simulink model "PosCtrl_tune"  (R2020b)
settings: Solver=FixedStepAuto  StartTime=0.0  StopTime=inf  FixedStep=0.01  RelTol=1e-3
InitFcn:
  | Init_control;
values from neighbouring files (symbols this model uses):
  DEG2RAD = 0.0174533    [Init_control.m]
  Kd_PITCH_AngleRate = 0.001    [Init_control.m]
  Kd_ROLL_AngleRate = 0.001    [Init_control.m]
  Kd_YAW_AngleRate = 0.00    (= 0)    [Init_control.m]
  Ki_PITCH_AngleRate = 0.02    [Init_control.m]
  Ki_ROLL_AngleRate = 0.02    [Init_control.m]
  Ki_YAW_AngleRate = 0.01    [Init_control.m]
  Kp_PITCH_ANGLE = 6.5    [Init_control.m]
  Kp_PITCH_AngleRate = 0.1    [Init_control.m]
  Kp_ROLL_ANGLE = 6.5    [Init_control.m]
  Kp_ROLL_AngleRate = 0.1    [Init_control.m]
  Kp_YAW_ANGLE = 3    [Init_control.m]
  Kp_YAW_AngleRate = 0.5    [Init_control.m]
  Kpxp = 1.0    (= 1)    [Init_control.m]
  Kpyp = 1.0    (= 1)    [Init_control.m]
  Kpzp = 4.0    (= 4)    [Init_control.m]
  Kvxd = 0.01    [Init_control.m]
  Kvxi = 0.4    [Init_control.m]
  Kvxp = 2.5    [Init_control.m]
  Kvyd = 0.01    [Init_control.m]
  Kvyi = 0.4    [Init_control.m]
  Kvyp = 2.5    [Init_control.m]
  Kvzd = 0.005    [Init_control.m]
  Kvzi = 0.01    [Init_control.m]
  Kvzp = 0.45    [Init_control.m]
  MAX_CONTROL_ANGLE_PITCH = 35    [Init_control.m]
  MAX_CONTROL_ANGLE_RATE_PITCH = 220    [Init_control.m]
  MAX_CONTROL_ANGLE_RATE_ROLL = 220    [Init_control.m]
  MAX_CONTROL_ANGLE_RATE_Y = 200    [Init_control.m]
  MAX_CONTROL_ANGLE_ROLL = 35    [Init_control.m]
  MAX_CONTROL_VELOCITY_XY = 17.6    [Init_control.m]
  MAX_CONTROL_VELOCITY_Z = 5    [Init_control.m]
  MAX_MAN_THR = 0.9    [Init_control.m]
  ModelInit_AngEuler = [0, 0, 0]    [Init_control.m]
  ModelInit_PosE0 = [0, 0, 0]    [Init_control.m]
  ModelInit_Rads = sqrt((ModelParam_uavMass*ModelParam_envGravityAcc)/(4*ModelParam_rotorCt))    [Init_control.m]
  ModelInit_RateB = [0, 0, 0]    [Init_control.m]
  ModelInit_VelB = [0, 0, 0]    [Init_control.m]
  Saturation_I_ah = 3.43    [Init_control.m]
  Saturation_I_az = 5    [Init_control.m]
  Saturation_I_RP_Max = 0.3    [Init_control.m]
  Saturation_I_RP_Min = -0.3    [Init_control.m]
  Saturation_I_Y_Max = 0.2    [Init_control.m]
  Saturation_I_Y_Min = -0.2    [Init_control.m]
  THR_HOVER = (ModelInit_Rads-ModelParam_motorWb)/ModelParam_motorCr    [Init_control.m]
undefined symbols (not defined in the file or in its folder): DiscIntNeverNeededParam, ModelParam_envGravityAcc, ModelParam_motorCr, ModelParam_motorJm, ModelParam_motorT, ModelParam_motorWb, ModelParam_rotorCm, ModelParam_rotorCt, ModelParam_uavCCm, ModelParam_uavCd, ModelParam_uavJ, ModelParam_uavMass, ModelParam_uavR
libraries: simulink x24, slrealtimeutilitieslib x8, sharedutil x8, dspnetwork x8, aerolibanimutils x1
(part 1 of 3)
settings Model: Creator=wsh  LastModifiedBy=chenjiaqing
settings DataIOCC: ReturnWorkspaceOutputs=off
settings DebuggingCC: BusObjectLabelMismatch=error  ArithmeticOperatorsInVariantConditions=warning
settings SFSimCC: SimUseLocalCustomCode=off  CustomCodeUndefinedFunction=UseInterfaceOnly
settings RTWCC: RTWUseLocalCustomCode=off
settings CodeAppCC: StateflowObjectComments=on

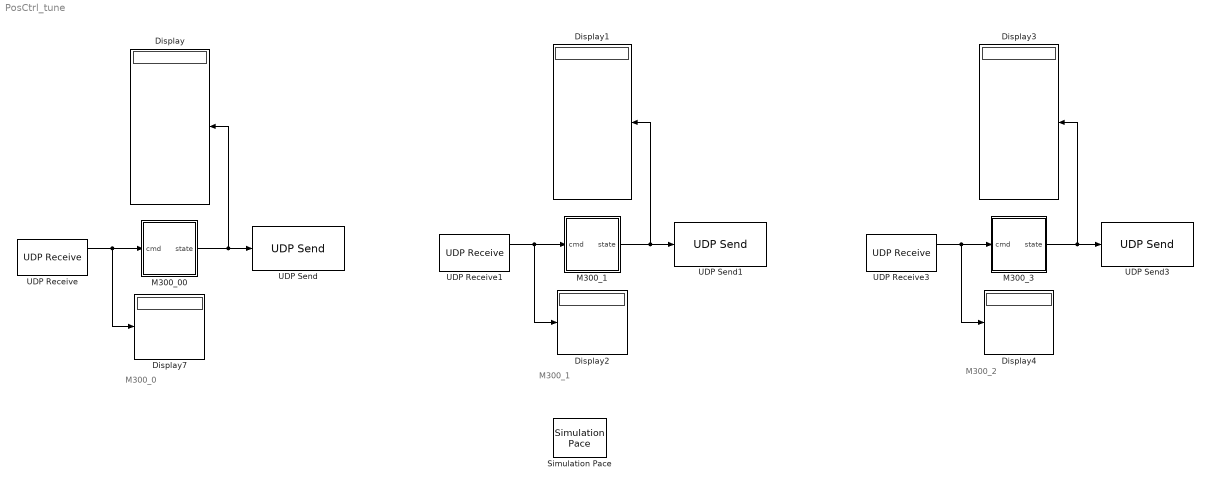
== system PosCtrl_tune ==
  note: M300_0
  note: M300_1
  note: M300_2
  Display{,1..4,7} (6 alike) : Display
      Display2 settings: Decimation=4
      Display4 settings: Decimation=4
      Display7 settings: Decimation=4
  M300_00 : Subsystem
  M300_1 : Subsystem
  M300_3 : Subsystem
  Simulation Pace : aerolibanimutils/Simulation Pace  SimulationPace=1  SleepMode=MATLAB Thread  OutputPaceError=off  SampleTime=-1
      settings: AttributesFormatString=%<SimulationPace> sec/sec
  UDP Receive : dspnetwork/UDP Receive  localURL='0.0.0.0'  localPort=udp_cmd0  remoteURL='127.0.0.1'  remotePort=-1  recvBufferSize=4  dims=4  signalDatatype=double  isComplex=off  isVarSize=off  showBlockingTime=off  blockingTime=0  sampletime=-1  blockPlatform=[]
  UDP Receive1 : dspnetwork/UDP Receive  localURL='0.0.0.0'  localPort=udp_cmd1  remoteURL='127.0.0.1'  remotePort=-1  recvBufferSize=4  dims=4  signalDatatype=double  isComplex=off  isVarSize=off  showBlockingTime=off  blockingTime=0  sampletime=-1  blockPlatform=[]
  UDP Receive3 : dspnetwork/UDP Receive  localURL='0.0.0.0'  localPort=udp_cmd2  remoteURL='127.0.0.1'  remotePort=-1  recvBufferSize=4  dims=4  signalDatatype=double  isComplex=off  isVarSize=off  showBlockingTime=off  blockingTime=0  sampletime=-1  blockPlatform=[]
  UDP Send : dspnetwork/UDP Send  remoteURL='127.0.0.1'  remotePort=udp_state0  localURL='0.0.0.0'  localPortSource=Automatically determine  localPort=25000  sendBufferSize=1  sampletime=-1  blockPlatform=[]  separateLengthPort=0
  UDP Send1 : dspnetwork/UDP Send  remoteURL='127.0.0.1'  remotePort=udp_state1  localURL='0.0.0.0'  localPortSource=Automatically determine  localPort=25000  sendBufferSize=1  sampletime=-1  blockPlatform=[]  separateLengthPort=0
  UDP Send3 : dspnetwork/UDP Send  remoteURL='127.0.0.1'  remotePort=udp_state2  localURL='0.0.0.0'  localPortSource=Automatically determine  localPort=25000  sendBufferSize=1  sampletime=-1  blockPlatform=[]  separateLengthPort=0
  wires:
  UDP Receive/1 -> Display7/1, M300_00/1(cmd)
  M300_00/1(state) -> UDP Send/1, Display/1
  UDP Receive1/1 -> Display2/1, M300_1/1(cmd)
  M300_1/1(state) -> UDP Send1/1, Display1/1
  UDP Receive3/1 -> Display4/1, M300_3/1(cmd)
  M300_3/1(state) -> UDP Send3/1, Display3/1

== system PosCtrl_tune/M300_00 ==
  cmd : Inport
  Byte Packing : slrealtimeutilitieslib/Byte Packing  MaskPackedDataType=double  MaskUnpackedDataTypes={'double','double','double','double','double','double','double','double','double','double'}  MaskAlignment=1
  Byte Unpacking : slrealtimeutilitieslib/Byte Unpacking  MaskUnpackedDataTypes={'double','double','double','double'}  MaskUnpackedDataSizes={[1],[1],[1],[1]}  MaskAlignment=1
      settings: SourceProductBaseCode=XP
  Constant : Constant  Value=0
  Control System : Subsystem
  Demux{,1..3,5..6} (6 alike) : Demux  Outputs=3
  Demux4 : Demux
  Quadcopter Dynamics : Subsystem
  Terminator{,1..5} (6 alike) : Terminator
  state : Outport
  wires:
  Quadcopter Dynamics/2(VelE) -> Demux5/1, Demux3/1  "VelE"
  Quadcopter Dynamics/4(AngRateB) -> Demux6/1, Demux/1  "AngRateB"
  Demux1/1 -> Byte Packing/4, Control System/11(roll)
  Demux2/1 -> Byte Packing/1, Control System/14(x)
  Demux1/2 -> Byte Packing/5, Control System/12(pitch)
  Demux1/3 -> Byte Packing/6, Control System/13(yaw)
  Demux4/2 -> Byte Packing/8
  Demux2/2 -> Control System/15(y), Byte Packing/2
  Constant/1 -> Control System/5(vxd), Control System/6(vyd), Control System/7(vzd)
  Quadcopter Dynamics/5(MotorRPMS) -> Demux4/1
  Demux2/3 -> Control System/16(z), Byte Packing/3
  Demux4/3 -> Byte Packing/7
  Quadcopter Dynamics/1(PosE) -> Demux2/1  "PosE"
  Demux4/4 -> Byte Packing/9
  Demux/3 -> Control System/10(r)
  Demux4/1 -> Byte Packing/10
  Quadcopter Dynamics/3(AngEuler) -> Demux1/1  "AngEular"
  Demux/1 -> Control System/8(p)
  Demux/2 -> Control System/9(q)
  Control System/1(PWM) -> Quadcopter Dynamics/1(inPWMs)
  Demux3/3 -> Control System/19(vz)
  Demux3/1 -> Control System/17(vx)
  Demux3/2 -> Control System/18(vy)
  cmd/1 -> Byte Unpacking/1
  Byte Packing/1 -> state/1
  Byte Unpacking/1 -> Control System/1(xd)
  Byte Unpacking/2 -> Control System/2(yd)
  Byte Unpacking/3 -> Control System/3(zd)
  Byte Unpacking/4 -> Control System/4(yaw_d)
  Demux5/1 -> Terminator/1
  Demux5/2 -> Terminator1/1
  Demux5/3 -> Terminator2/1
  Demux6/3 -> Terminator5/1
  Demux6/1 -> Terminator3/1
  Demux6/2 -> Terminator4/1

== system PosCtrl_tune/M300_1 ==
  cmd : Inport
  Byte Packing : slrealtimeutilitieslib/Byte Packing  MaskPackedDataType=double  MaskUnpackedDataTypes={'double','double','double','double','double','double','double','double','double','double'}  MaskAlignment=1
  Byte Unpacking : slrealtimeutilitieslib/Byte Unpacking  MaskUnpackedDataTypes={'double','double','double','double'}  MaskUnpackedDataSizes={[1],[1],[1],[1]}  MaskAlignment=1
      settings: SourceProductBaseCode=XP
  Constant : Constant  Value=0
  Control System : Subsystem
  Demux{,1..3,5..6} (6 alike) : Demux  Outputs=3
  Demux4 : Demux
  Quadcopter Dynamics : Subsystem
  Terminator{,1..5} (6 alike) : Terminator
  state : Outport
  wires:
  Quadcopter Dynamics/2(VelE) -> Demux5/1, Demux3/1  "VelE"
  Quadcopter Dynamics/4(AngRateB) -> Demux6/1, Demux/1  "AngRateB"
  Demux1/1 -> Byte Packing/4, Control System/11(roll)
  Demux2/1 -> Byte Packing/1, Control System/14(x)
  Demux1/2 -> Byte Packing/5, Control System/12(pitch)
  Demux1/3 -> Byte Packing/6, Control System/13(yaw)
  Demux4/2 -> Byte Packing/8
  Demux2/2 -> Control System/15(y), Byte Packing/2
  Constant/1 -> Control System/5(vxd), Control System/6(vyd), Control System/7(vzd)
  Quadcopter Dynamics/5(MotorRPMS) -> Demux4/1
  Demux2/3 -> Control System/16(z), Byte Packing/3
  Demux4/3 -> Byte Packing/7
  Quadcopter Dynamics/1(PosE) -> Demux2/1  "PosE"
  Demux4/4 -> Byte Packing/9
  Demux/3 -> Control System/10(r)
  Demux4/1 -> Byte Packing/10
  Quadcopter Dynamics/3(AngEuler) -> Demux1/1  "AngEular"
  Demux/1 -> Control System/8(p)
  Demux/2 -> Control System/9(q)
  Control System/1(PWM) -> Quadcopter Dynamics/1(inPWMs)
  Demux3/3 -> Control System/19(vz)
  Demux3/1 -> Control System/17(vx)
  Demux3/2 -> Control System/18(vy)
  cmd/1 -> Byte Unpacking/1
  Byte Packing/1 -> state/1
  Byte Unpacking/1 -> Control System/1(xd)
  Byte Unpacking/2 -> Control System/2(yd)
  Byte Unpacking/3 -> Control System/3(zd)
  Byte Unpacking/4 -> Control System/4(yaw_d)
  Demux5/1 -> Terminator/1
  Demux5/2 -> Terminator1/1
  Demux5/3 -> Terminator2/1
  Demux6/3 -> Terminator5/1
  Demux6/1 -> Terminator3/1
  Demux6/2 -> Terminator4/1

== system PosCtrl_tune/M300_3 ==
  cmd : Inport
  Byte Packing : slrealtimeutilitieslib/Byte Packing  MaskPackedDataType=double  MaskUnpackedDataTypes={'double','double','double','double','double','double','double','double','double','double'}  MaskAlignment=1
  Byte Unpacking : slrealtimeutilitieslib/Byte Unpacking  MaskUnpackedDataTypes={'double','double','double','double'}  MaskUnpackedDataSizes={[1],[1],[1],[1]}  MaskAlignment=1
      settings: SourceProductBaseCode=XP
  Constant : Constant  Value=0
  Control System : Subsystem
  Demux{,1..3,5..6} (6 alike) : Demux  Outputs=3
  Demux4 : Demux
  M300_2 : Subsystem  Commented=on
  Quadcopter Dynamics : Subsystem
  Terminator{,1..5} (6 alike) : Terminator
  UDP Receive2 : dspnetwork/UDP Receive  Commented=on  localURL='0.0.0.0'  localPort=udp_cmd2  remoteURL='127.0.0.1'  remotePort=-1  recvBufferSize=4  dims=4  signalDatatype=double  isComplex=off  isVarSize=off  showBlockingTime=off  blockingTime=0  sampletime=-1  blockPlatform=[]
  UDP Send2 : dspnetwork/UDP Send  Commented=on  remoteURL='127.0.0.1'  remotePort=udp_state2  localURL='0.0.0.0'  localPortSource=Automatically determine  localPort=25000  sendBufferSize=1  sampletime=-1  blockPlatform=[]  separateLengthPort=0
  state : Outport
  wires:
  Quadcopter Dynamics/2(VelE) -> Demux5/1, Demux3/1  "VelE"
  Quadcopter Dynamics/4(AngRateB) -> Demux6/1, Demux/1  "AngRateB"
  Demux1/1 -> Byte Packing/4, Control System/11(roll)
  Demux2/1 -> Byte Packing/1, Control System/14(x)
  Demux1/2 -> Byte Packing/5, Control System/12(pitch)
  Demux1/3 -> Byte Packing/6, Control System/13(yaw)
  Demux4/2 -> Byte Packing/8
  Demux2/2 -> Control System/15(y), Byte Packing/2
  Constant/1 -> Control System/5(vxd), Control System/6(vyd), Control System/7(vzd)
  Quadcopter Dynamics/5(MotorRPMS) -> Demux4/1
  Demux2/3 -> Control System/16(z), Byte Packing/3
  Demux4/3 -> Byte Packing/7
  Quadcopter Dynamics/1(PosE) -> Demux2/1  "PosE"
  Demux4/4 -> Byte Packing/9
  Demux/3 -> Control System/10(r)
  Demux4/1 -> Byte Packing/10
  Quadcopter Dynamics/3(AngEuler) -> Demux1/1  "AngEular"
  Demux/1 -> Control System/8(p)
  Demux/2 -> Control System/9(q)
  Control System/1(PWM) -> Quadcopter Dynamics/1(inPWMs)
  Demux3/3 -> Control System/19(vz)
  Demux3/1 -> Control System/17(vx)
  Demux3/2 -> Control System/18(vy)
  cmd/1 -> Byte Unpacking/1
  Byte Packing/1 -> state/1
  Byte Unpacking/1 -> Control System/1(xd)
  Byte Unpacking/2 -> Control System/2(yd)
  Byte Unpacking/3 -> Control System/3(zd)
  Byte Unpacking/4 -> Control System/4(yaw_d)
  Demux5/1 -> Terminator/1
  Demux5/2 -> Terminator1/1
  Demux5/3 -> Terminator2/1
  Demux6/3 -> Terminator5/1
  Demux6/1 -> Terminator3/1
  Demux6/2 -> Terminator4/1
  M300_2/1(state) -> UDP Send2/1
  UDP Receive2/1 -> M300_2/1(cmd)

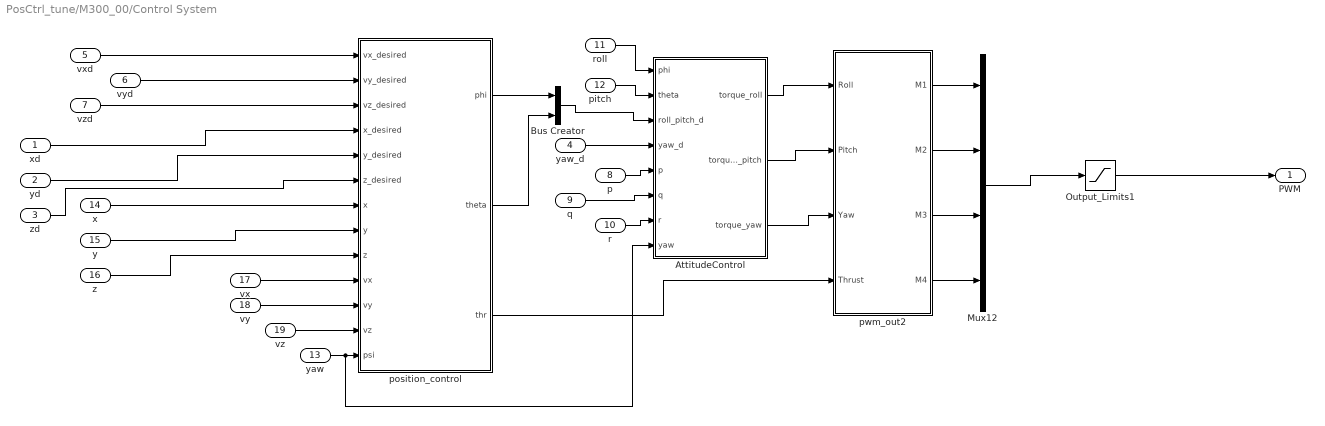
== system PosCtrl_tune/M300_00/Control System ==
  xd : Inport
  yd : Inport  Port=2
  zd : Inport  Port=3
  yaw_d : Inport  Port=4
  vxd : Inport  Port=5
  vyd : Inport  Port=6
  vzd : Inport  Port=7
  p : Inport  Port=8  PortDimensions=1
  q : Inport  Port=9  PortDimensions=1
  r : Inport  Port=10  PortDimensions=1
  roll : Inport  Port=11  PortDimensions=1
  pitch : Inport  Port=12  PortDimensions=1
  yaw : Inport  Port=13  PortDimensions=1
  x : Inport  Port=14
  y : Inport  Port=15
  z : Inport  Port=16
  vx : Inport  Port=17
  vy : Inport  Port=18
  vz : Inport  Port=19
  AttitudeControl : Subsystem
  Bus Creator : BusCreator  Inputs=2
  Mux12 : Mux
  Output_Limits1 : Saturate  UpperLimit=2000  LowerLimit=1000
  position_control : Subsystem
  pwm_out2 : MATLAB Function  SystemSampleTime=0.004
  PWM : Outport  VectorParamsAs1DForOutWhenUnconnected=off
  wires:
  Mux12/1 -> Output_Limits1/1
  AttitudeControl/2(torque_pitch) -> pwm_out2/2(Pitch)
  AttitudeControl/1(torque_roll) -> pwm_out2/1(Roll)
  pwm_out2/1(M1) -> Mux12/1
  pwm_out2/3(M3) -> Mux12/3
  pwm_out2/2(M2) -> Mux12/2
  AttitudeControl/3(torque_yaw) -> pwm_out2/3(Yaw)
  yaw_d/1 -> AttitudeControl/4(yaw_d)
  p/1 -> AttitudeControl/5(p)
  pwm_out2/4(M4) -> Mux12/4
  roll/1 -> AttitudeControl/1(phi)
  pitch/1 -> AttitudeControl/2(theta)
  position_control/1(phi) -> Bus Creator/1
  position_control/2(theta) -> Bus Creator/2
  Bus Creator/1 -> AttitudeControl/3(roll_pitch_d)
  position_control/3(thr) -> pwm_out2/4(Thrust)
  vxd/1 -> position_control/1(vx_desired)
  vyd/1 -> position_control/2(vy_desired)
  vzd/1 -> position_control/3(vz_desired)
  x/1 -> position_control/7(x)
  y/1 -> position_control/8(y)
  z/1 -> position_control/9(z)
  vx/1 -> position_control/10(vx)
  vy/1 -> position_control/11(vy)
  vz/1 -> position_control/12(vz)
  yaw/1 -> AttitudeControl/8(yaw), position_control/13(psi)
  Output_Limits1/1 -> PWM/1
  r/1 -> AttitudeControl/7(r)
  q/1 -> AttitudeControl/6(q)
  xd/1 -> position_control/4(x_desired)
  yd/1 -> position_control/5(y_desired)
  zd/1 -> position_control/6(z_desired)

== system PosCtrl_tune/M300_00/Quadcopter Dynamics ==
  note: 输入为1000至2000的PWM信号，
      | 需要归一化为0~1。
  inPWMs : Inport
  Constant2 : Constant  Value=[1000,1000,1000,1000]
  Demux2 : Demux
  Gain : Gain  Gain=30/pi
  Gain1 : Gain  Gain=1/1000
  Gain2 : Gain  Gain=-1
  Gain3 : Gain  Gain=10
  Gain4 : Gain  Gain=-1
  Gain5 : Gain
  Gain6 : Gain
  Mux : Mux
  Product1 : Product
  Saturation : Saturate  UpperLimit=1  LowerLimit=0
  Sum : Sum  Inputs=|+-
  g : Constant  Value=[0,0,ModelParam_envGravityAcc]
  mass : Constant  Value=ModelParam_uavMass
  六自由度模型 : Subsystem
  控制效果模型 : Subsystem
  电机动态模型 : Subsystem
  PosE : Outport  VectorParamsAs1DForOutWhenUnconnected=off
  VelE : Outport  Port=2  VectorParamsAs1DForOutWhenUnconnected=off
  AngEuler : Outport  Port=3  VectorParamsAs1DForOutWhenUnconnected=off
  AngRateB : Outport  Port=4  VectorParamsAs1DForOutWhenUnconnected=off
  MotorRPMS : Outport  Port=5  VectorParamsAs1DForOutWhenUnconnected=off
  wires:
  Saturation/1 -> 电机动态模型/1(inPWMs)
  六自由度模型/6("p,q,r ") -> 控制效果模型/5(p.q,r), AngRateB/1
  mass/1 -> Product1/1
  六自由度模型/4(DCM) -> 控制效果模型/3(DCM)
  电机动态模型/1(MotorRads) -> Gain/1, 控制效果模型/1(MotorRads)
  Gain1/1 -> Saturation/1
  六自由度模型/2(ve) -> VelE/1
  Sum/1 -> Gain1/1
  Product1/1 -> 控制效果模型/2(mg)
  六自由度模型/5("vb ") -> 控制效果模型/4(Vb)
  六自由度模型/1("xe ") -> PosE/1
  六自由度模型/3(Euler) -> AngEuler/1
  控制效果模型/1(Mb) -> 六自由度模型/1(Mb)
  inPWMs/1 -> Sum/1
  控制效果模型/2(Fb) -> 六自由度模型/2(f)
  Constant2/1 -> Sum/2
  g/1 -> Product1/2
  Demux2/3 -> Gain4/1
  Demux2/4 -> Gain6/1
  Gain2/1 -> Mux/1
  Gain4/1 -> Mux/3
  Gain6/1 -> Mux/4
  Mux/1 -> Gain3/1
  Demux2/1 -> Gain2/1
  Gain5/1 -> Mux/2
  Demux2/2 -> Gain5/1
  Gain/1 -> Demux2/1
  Gain3/1 -> MotorRPMS/1

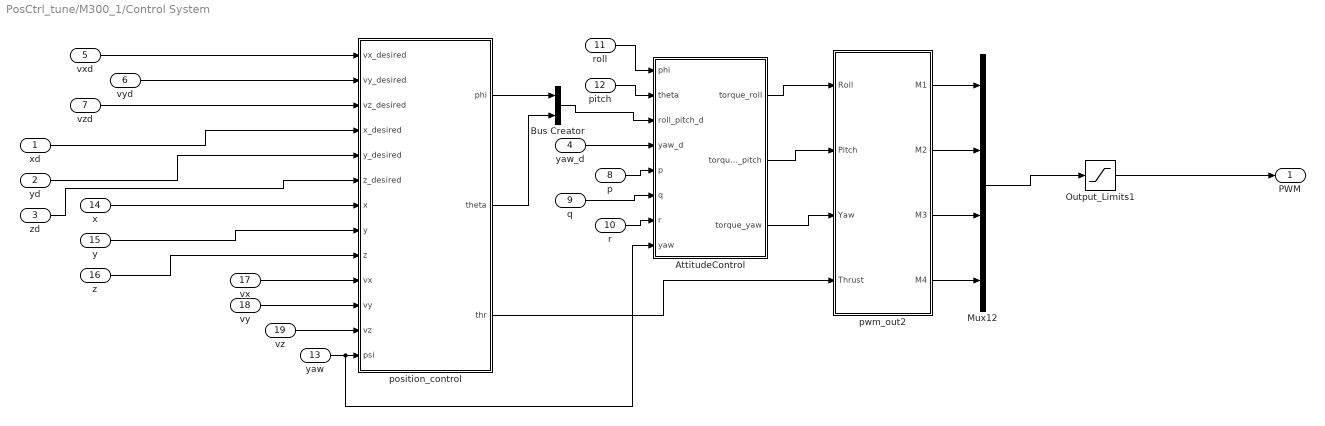
== system PosCtrl_tune/M300_1/Control System ==
  xd : Inport
  yd : Inport  Port=2
  zd : Inport  Port=3
  yaw_d : Inport  Port=4
  vxd : Inport  Port=5
  vyd : Inport  Port=6
  vzd : Inport  Port=7
  p : Inport  Port=8  PortDimensions=1
  q : Inport  Port=9  PortDimensions=1
  r : Inport  Port=10  PortDimensions=1
  roll : Inport  Port=11  PortDimensions=1
  pitch : Inport  Port=12  PortDimensions=1
  yaw : Inport  Port=13  PortDimensions=1
  x : Inport  Port=14
  y : Inport  Port=15
  z : Inport  Port=16
  vx : Inport  Port=17
  vy : Inport  Port=18
  vz : Inport  Port=19
  AttitudeControl : Subsystem
  Bus Creator : BusCreator  Inputs=2
  Mux12 : Mux
  Output_Limits1 : Saturate  UpperLimit=2000  LowerLimit=1000
  position_control : Subsystem
  pwm_out2 : MATLAB Function  SystemSampleTime=0.004
  PWM : Outport  VectorParamsAs1DForOutWhenUnconnected=off
  wires:
  Mux12/1 -> Output_Limits1/1
  AttitudeControl/2(torque_pitch) -> pwm_out2/2(Pitch)
  AttitudeControl/1(torque_roll) -> pwm_out2/1(Roll)
  pwm_out2/1(M1) -> Mux12/1
  pwm_out2/3(M3) -> Mux12/3
  pwm_out2/2(M2) -> Mux12/2
  AttitudeControl/3(torque_yaw) -> pwm_out2/3(Yaw)
  yaw_d/1 -> AttitudeControl/4(yaw_d)
  p/1 -> AttitudeControl/5(p)
  pwm_out2/4(M4) -> Mux12/4
  roll/1 -> AttitudeControl/1(phi)
  pitch/1 -> AttitudeControl/2(theta)
  position_control/1(phi) -> Bus Creator/1
  position_control/2(theta) -> Bus Creator/2
  Bus Creator/1 -> AttitudeControl/3(roll_pitch_d)
  position_control/3(thr) -> pwm_out2/4(Thrust)
  vxd/1 -> position_control/1(vx_desired)
  vyd/1 -> position_control/2(vy_desired)
  vzd/1 -> position_control/3(vz_desired)
  x/1 -> position_control/7(x)
  y/1 -> position_control/8(y)
  z/1 -> position_control/9(z)
  vx/1 -> position_control/10(vx)
  vy/1 -> position_control/11(vy)
  vz/1 -> position_control/12(vz)
  yaw/1 -> AttitudeControl/8(yaw), position_control/13(psi)
  Output_Limits1/1 -> PWM/1
  r/1 -> AttitudeControl/7(r)
  q/1 -> AttitudeControl/6(q)
  xd/1 -> position_control/4(x_desired)
  yd/1 -> position_control/5(y_desired)
  zd/1 -> position_control/6(z_desired)

== system PosCtrl_tune/M300_1/Quadcopter Dynamics ==
  note: 输入为1000至2000的PWM信号，
      | 需要归一化为0~1。
  inPWMs : Inport
  Constant2 : Constant  Value=[1000,1000,1000,1000]
  Demux2 : Demux
  Gain : Gain  Gain=30/pi
  Gain1 : Gain  Gain=1/1000
  Gain2 : Gain  Gain=-1
  Gain3 : Gain  Gain=10
  Gain4 : Gain  Gain=-1
  Gain5 : Gain
  Gain6 : Gain
  Mux : Mux
  Product1 : Product
  Saturation : Saturate  UpperLimit=1  LowerLimit=0
  Sum : Sum  Inputs=|+-
  g : Constant  Value=[0,0,ModelParam_envGravityAcc]
  mass : Constant  Value=ModelParam_uavMass
  六自由度模型 : Subsystem
  控制效果模型 : Subsystem
  电机动态模型 : Subsystem
  PosE : Outport  VectorParamsAs1DForOutWhenUnconnected=off
  VelE : Outport  Port=2  VectorParamsAs1DForOutWhenUnconnected=off
  AngEuler : Outport  Port=3  VectorParamsAs1DForOutWhenUnconnected=off
  AngRateB : Outport  Port=4  VectorParamsAs1DForOutWhenUnconnected=off
  MotorRPMS : Outport  Port=5  VectorParamsAs1DForOutWhenUnconnected=off
  wires:
  Saturation/1 -> 电机动态模型/1(inPWMs)
  六自由度模型/6("p,q,r ") -> 控制效果模型/5(p.q,r), AngRateB/1
  mass/1 -> Product1/1
  六自由度模型/4(DCM) -> 控制效果模型/3(DCM)
  电机动态模型/1(MotorRads) -> Gain/1, 控制效果模型/1(MotorRads)
  Gain1/1 -> Saturation/1
  六自由度模型/2(ve) -> VelE/1
  Sum/1 -> Gain1/1
  Product1/1 -> 控制效果模型/2(mg)
  六自由度模型/5("vb ") -> 控制效果模型/4(Vb)
  六自由度模型/1("xe ") -> PosE/1
  六自由度模型/3(Euler) -> AngEuler/1
  控制效果模型/1(Mb) -> 六自由度模型/1(Mb)
  inPWMs/1 -> Sum/1
  控制效果模型/2(Fb) -> 六自由度模型/2(f)
  Constant2/1 -> Sum/2
  g/1 -> Product1/2
  Demux2/3 -> Gain4/1
  Demux2/4 -> Gain6/1
  Gain2/1 -> Mux/1
  Gain4/1 -> Mux/3
  Gain6/1 -> Mux/4
  Mux/1 -> Gain3/1
  Demux2/1 -> Gain2/1
  Gain5/1 -> Mux/2
  Demux2/2 -> Gain5/1
  Gain/1 -> Demux2/1
  Gain3/1 -> MotorRPMS/1

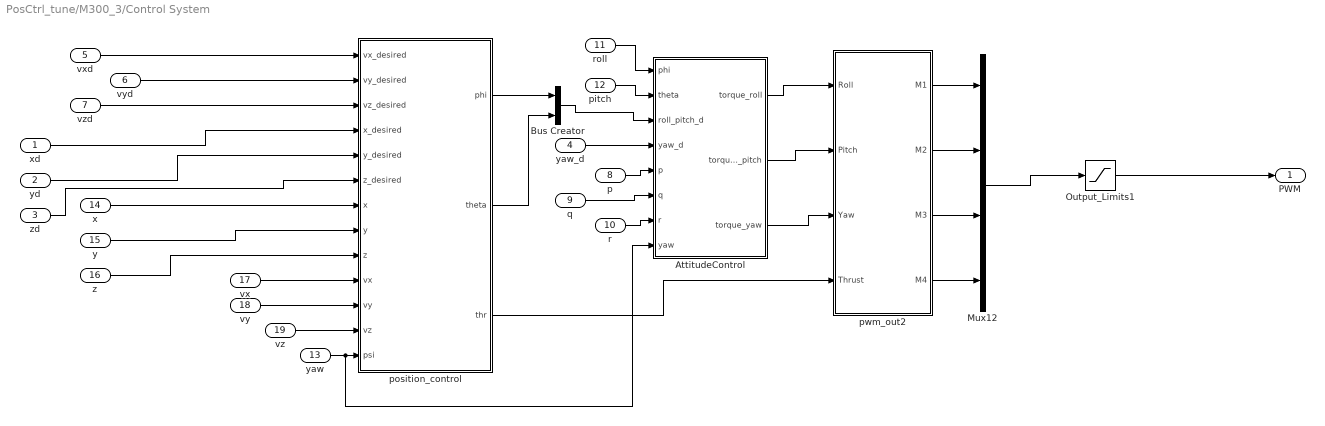
== system PosCtrl_tune/M300_3/Control System ==
  xd : Inport
  yd : Inport  Port=2
  zd : Inport  Port=3
  yaw_d : Inport  Port=4
  vxd : Inport  Port=5
  vyd : Inport  Port=6
  vzd : Inport  Port=7
  p : Inport  Port=8  PortDimensions=1
  q : Inport  Port=9  PortDimensions=1
  r : Inport  Port=10  PortDimensions=1
  roll : Inport  Port=11  PortDimensions=1
  pitch : Inport  Port=12  PortDimensions=1
  yaw : Inport  Port=13  PortDimensions=1
  x : Inport  Port=14
  y : Inport  Port=15
  z : Inport  Port=16
  vx : Inport  Port=17
  vy : Inport  Port=18
  vz : Inport  Port=19
  AttitudeControl : Subsystem
  Bus Creator : BusCreator  Inputs=2
  Mux12 : Mux
  Output_Limits1 : Saturate  UpperLimit=2000  LowerLimit=1000
  position_control : Subsystem
  pwm_out2 : MATLAB Function  SystemSampleTime=0.004
  PWM : Outport  VectorParamsAs1DForOutWhenUnconnected=off
  wires:
  Mux12/1 -> Output_Limits1/1
  AttitudeControl/2(torque_pitch) -> pwm_out2/2(Pitch)
  AttitudeControl/1(torque_roll) -> pwm_out2/1(Roll)
  pwm_out2/1(M1) -> Mux12/1
  pwm_out2/3(M3) -> Mux12/3
  pwm_out2/2(M2) -> Mux12/2
  AttitudeControl/3(torque_yaw) -> pwm_out2/3(Yaw)
  yaw_d/1 -> AttitudeControl/4(yaw_d)
  p/1 -> AttitudeControl/5(p)
  pwm_out2/4(M4) -> Mux12/4
  roll/1 -> AttitudeControl/1(phi)
  pitch/1 -> AttitudeControl/2(theta)
  position_control/1(phi) -> Bus Creator/1
  position_control/2(theta) -> Bus Creator/2
  Bus Creator/1 -> AttitudeControl/3(roll_pitch_d)
  position_control/3(thr) -> pwm_out2/4(Thrust)
  vxd/1 -> position_control/1(vx_desired)
  vyd/1 -> position_control/2(vy_desired)
  vzd/1 -> position_control/3(vz_desired)
  x/1 -> position_control/7(x)
  y/1 -> position_control/8(y)
  z/1 -> position_control/9(z)
  vx/1 -> position_control/10(vx)
  vy/1 -> position_control/11(vy)
  vz/1 -> position_control/12(vz)
  yaw/1 -> AttitudeControl/8(yaw), position_control/13(psi)
  Output_Limits1/1 -> PWM/1
  r/1 -> AttitudeControl/7(r)
  q/1 -> AttitudeControl/6(q)
  xd/1 -> position_control/4(x_desired)
  yd/1 -> position_control/5(y_desired)
  zd/1 -> position_control/6(z_desired)

== system PosCtrl_tune/M300_3/M300_2 ==
  cmd : Inport
  Byte Packing : slrealtimeutilitieslib/Byte Packing  MaskPackedDataType=double  MaskUnpackedDataTypes={'double','double','double','double','double','double','double','double','double','double'}  MaskAlignment=1
  Byte Unpacking : slrealtimeutilitieslib/Byte Unpacking  MaskUnpackedDataTypes={'double','double','double','double'}  MaskUnpackedDataSizes={[1],[1],[1],[1]}  MaskAlignment=1
      settings: SourceProductBaseCode=XP
  Constant : Constant  Value=0
  Control System : Subsystem
  Demux{,1..3} (4 alike) : Demux  Outputs=3
  Demux4 : Demux
  Quadcopter Dynamics : Subsystem
  state : Outport
  wires:
  Quadcopter Dynamics/2(VelE) -> Demux3/1  "VelE"
  Quadcopter Dynamics/4(AngRateB) -> Demux/1  "AngRateB"
  Demux1/1 -> Byte Packing/4, Control System/11(roll)
  Demux2/1 -> Byte Packing/1, Control System/14(x)
  Byte Unpacking/1 -> Control System/1(xd)
  Demux1/2 -> Byte Packing/5, Control System/12(pitch)
  Demux1/3 -> Byte Packing/6, Control System/13(yaw)
  Demux4/2 -> Byte Packing/8
  Demux2/2 -> Control System/15(y), Byte Packing/2
  Constant/1 -> Control System/5(vxd), Control System/6(vyd), Control System/7(vzd)
  Byte Unpacking/2 -> Control System/2(yd)
  Quadcopter Dynamics/5(MotorRPMS) -> Demux4/1
  Demux2/3 -> Control System/16(z), Byte Packing/3
  Demux4/3 -> Byte Packing/7
  Quadcopter Dynamics/1(PosE) -> Demux2/1  "PosE"
  Demux4/4 -> Byte Packing/9
  Demux/3 -> Control System/10(r)
  Demux4/1 -> Byte Packing/10
  Byte Unpacking/3 -> Control System/3(zd)
  Quadcopter Dynamics/3(AngEuler) -> Demux1/1  "AngEular"
  Demux/1 -> Control System/8(p)
  Demux/2 -> Control System/9(q)
  Control System/1(PWM) -> Quadcopter Dynamics/1(inPWMs)
  Demux3/3 -> Control System/19(vz)
  Demux3/1 -> Control System/17(vx)
  Demux3/2 -> Control System/18(vy)
  cmd/1 -> Byte Unpacking/1
  Byte Packing/1 -> state/1
  Byte Unpacking/4 -> Control System/4(yawRate_d)

== system PosCtrl_tune/M300_3/Quadcopter Dynamics ==
  note: 输入为1000至2000的PWM信号，
      | 需要归一化为0~1。
  inPWMs : Inport
  Constant2 : Constant  Value=[1000,1000,1000,1000]
  Demux2 : Demux
  Gain : Gain  Gain=30/pi
  Gain1 : Gain  Gain=1/1000
  Gain2 : Gain  Gain=-1
  Gain3 : Gain  Gain=10
  Gain4 : Gain  Gain=-1
  Gain5 : Gain
  Gain6 : Gain
  Mux : Mux
  Product1 : Product
  Saturation : Saturate  UpperLimit=1  LowerLimit=0
  Sum : Sum  Inputs=|+-
  g : Constant  Value=[0,0,ModelParam_envGravityAcc]
  mass : Constant  Value=ModelParam_uavMass
  六自由度模型 : Subsystem
  控制效果模型 : Subsystem
  电机动态模型 : Subsystem
  PosE : Outport  VectorParamsAs1DForOutWhenUnconnected=off
  VelE : Outport  Port=2  VectorParamsAs1DForOutWhenUnconnected=off
  AngEuler : Outport  Port=3  VectorParamsAs1DForOutWhenUnconnected=off
  AngRateB : Outport  Port=4  VectorParamsAs1DForOutWhenUnconnected=off
  MotorRPMS : Outport  Port=5  VectorParamsAs1DForOutWhenUnconnected=off
  wires:
  Saturation/1 -> 电机动态模型/1(inPWMs)
  六自由度模型/6("p,q,r ") -> 控制效果模型/5(p.q,r), AngRateB/1
  mass/1 -> Product1/1
  六自由度模型/4(DCM) -> 控制效果模型/3(DCM)
  电机动态模型/1(MotorRads) -> Gain/1, 控制效果模型/1(MotorRads)
  Gain1/1 -> Saturation/1
  六自由度模型/2(ve) -> VelE/1
  Sum/1 -> Gain1/1
  Product1/1 -> 控制效果模型/2(mg)
  六自由度模型/5("vb ") -> 控制效果模型/4(Vb)
  六自由度模型/1("xe ") -> PosE/1
  六自由度模型/3(Euler) -> AngEuler/1
  控制效果模型/1(Mb) -> 六自由度模型/1(Mb)
  inPWMs/1 -> Sum/1
  控制效果模型/2(Fb) -> 六自由度模型/2(f)
  Constant2/1 -> Sum/2
  g/1 -> Product1/2
  Demux2/3 -> Gain4/1
  Demux2/4 -> Gain6/1
  Gain2/1 -> Mux/1
  Gain4/1 -> Mux/3
  Gain6/1 -> Mux/4
  Mux/1 -> Gain3/1
  Demux2/1 -> Gain2/1
  Gain5/1 -> Mux/2
  Demux2/2 -> Gain5/1
  Gain/1 -> Demux2/1
  Gain3/1 -> MotorRPMS/1

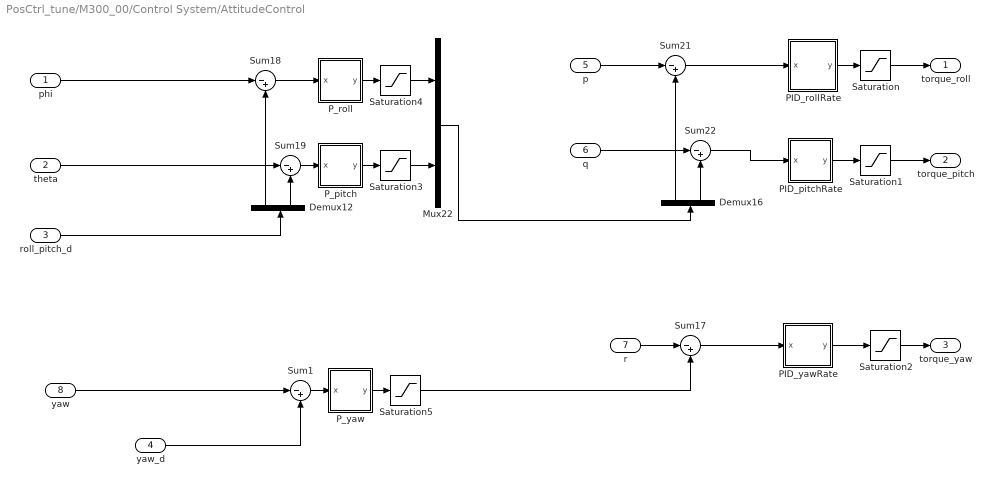
== system PosCtrl_tune/M300_00/Control System/AttitudeControl ==
  phi : Inport
  theta : Inport  Port=2
  roll_pitch_d : Inport  Port=3
  yaw_d : Inport  Port=4
  p : Inport  Port=5
  q : Inport  Port=6
  r : Inport  Port=7
  yaw : Inport  Port=8
  Demux12 : Demux  Outputs=2
  Demux16 : Demux  Outputs=2
  Mux22 : Mux  Inputs=2
  PID_pitchRate : Subsystem
  PID_rollRate : Subsystem
  PID_yawRate : Subsystem
  "P_pitch " : Subsystem
  "P_roll " : Subsystem
  P_yaw : Subsystem
  Saturation : Saturate  UpperLimit=1  LowerLimit=-1
  Saturation1 : Saturate  UpperLimit=1  LowerLimit=-1
  Saturation2 : Saturate
  Saturation3 : Saturate  UpperLimit=MAX_CONTROL_ANGLE_RATE_PITCH  LowerLimit=-MAX_CONTROL_ANGLE_RATE_PITCH
  Saturation4 : Saturate  UpperLimit=MAX_CONTROL_ANGLE_RATE_ROLL  LowerLimit=-MAX_CONTROL_ANGLE_RATE_ROLL
  Saturation5 : Saturate  UpperLimit=MAX_CONTROL_ANGLE_RATE_Y  LowerLimit=-MAX_CONTROL_ANGLE_RATE_Y
  Sum{1,17..19,21..22} (6 alike) : Sum  Inputs=|-+
  torque_roll : Outport  VectorParamsAs1DForOutWhenUnconnected=off
  torque_pitch : Outport  Port=2  VectorParamsAs1DForOutWhenUnconnected=off
  torque_yaw : Outport  Port=3  VectorParamsAs1DForOutWhenUnconnected=off
  wires:
  r/1 -> Sum17/1
  Sum19/1 -> "P_pitch "/1(x)
  "P_pitch "/1(y) -> Saturation3/1
  "P_roll "/1(y) -> Saturation4/1
  roll_pitch_d/1 -> Demux12/1
  Demux12/1 -> Sum18/2
  Demux12/2 -> Sum19/2
  phi/1 -> Sum18/1
  theta/1 -> Sum19/1
  Sum18/1 -> "P_roll "/1(x)
  Sum22/1 -> PID_pitchRate/1(x)
  Sum17/1 -> PID_yawRate/1(x)
  p/1 -> Sum21/1
  q/1 -> Sum22/1
  Sum21/1 -> PID_rollRate/1(x)
  Demux16/1 -> Sum21/2
  PID_pitchRate/1(y) -> Saturation1/1
  PID_rollRate/1(y) -> Saturation/1
  PID_yawRate/1(y) -> Saturation2/1
  Saturation/1 -> torque_roll/1
  Saturation1/1 -> torque_pitch/1
  Saturation2/1 -> torque_yaw/1
  Mux22/1 -> Demux16/1
  Saturation4/1 -> Mux22/1
  Saturation3/1 -> Mux22/2
  Demux16/2 -> Sum22/2
  Saturation5/1 -> Sum17/2
  Sum1/1 -> P_yaw/1(x)
  P_yaw/1(y) -> Saturation5/1
  yaw/1 -> Sum1/1
  yaw_d/1 -> Sum1/2

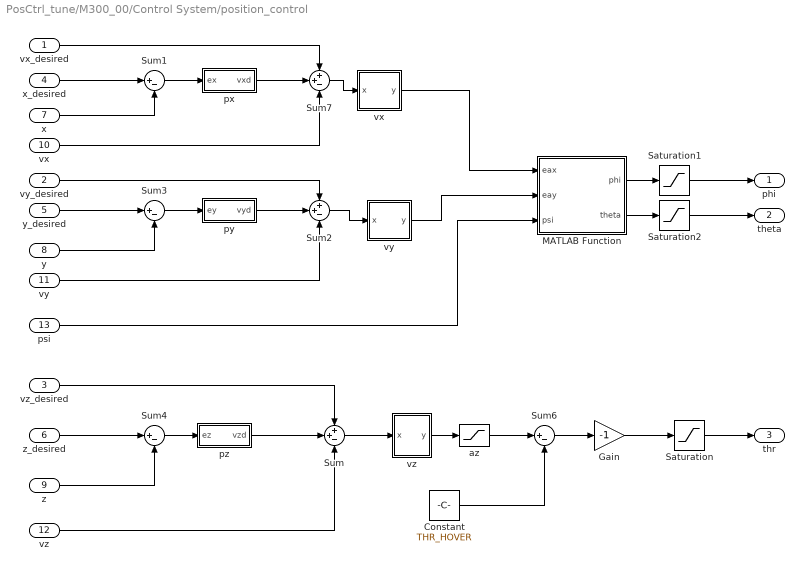
== system PosCtrl_tune/M300_00/Control System/position_control ==
  vx_desired : Inport
  vy_desired : Inport  Port=2
  vz_desired : Inport  Port=3
  x_desired : Inport  Port=4
  y_desired : Inport  Port=5
  z_desired : Inport  Port=6
  x : Inport  Port=7
  y : Inport  Port=8
  z : Inport  Port=9
  vx : Inport  Port=10
  vy : Inport  Port=11
  vz : Inport  Port=12
  psi : Inport  Port=13
  Constant : Constant  Value=THR_HOVER
  Gain : Gain  Gain=-1
  MATLAB Function : MATLAB Function  TreatAsAtomicUnit=on
  Saturation : Saturate  UpperLimit=MAX_MAN_THR  LowerLimit=0
  Saturation1 : Saturate  UpperLimit=MAX_CONTROL_ANGLE_ROLL*DEG2RAD  LowerLimit=-MAX_CONTROL_ANGLE_ROLL*DEG2RAD
  Saturation2 : Saturate  UpperLimit=MAX_CONTROL_ANGLE_PITCH*DEG2RAD  LowerLimit=-MAX_CONTROL_ANGLE_PITCH*DEG2RAD
  Sum : Sum  Inputs=++-
  Sum{1,3..4,6} (4 alike) : Sum  Inputs=|+-
  Sum2 : Sum  Inputs=++-
  Sum7 : Sum  Inputs=++-
  az : Saturate  UpperLimit=0.4  LowerLimit=-0.4
  px : Subsystem
  py : Subsystem
  pz : Subsystem
  "vx " : Subsystem
  "vy " : Subsystem
  "vz " : Subsystem
  phi : Outport  VectorParamsAs1DForOutWhenUnconnected=off
  theta : Outport  Port=2  VectorParamsAs1DForOutWhenUnconnected=off
  thr : Outport  Port=3  VectorParamsAs1DForOutWhenUnconnected=off
  wires:
  Saturation/1 -> thr/1
  Gain/1 -> Saturation/1
  Sum6/1 -> Gain/1
  "vz "/1(y) -> az/1
  Sum4/1 -> pz/1(ez)
  z/1 -> Sum4/2
  Constant/1 -> Sum6/2
  Sum/1 -> "vz "/1(x)
  vz/1 -> Sum/3
  x/1 -> Sum1/2
  y/1 -> Sum3/2
  Sum3/1 -> py/1(ey)
  y_desired/1 -> Sum3/1
  vy/1 -> Sum2/3
  Sum2/1 -> "vy "/1(x)
  Sum7/1 -> "vx "/1(x)
  Sum1/1 -> px/1(ex)
  vy_desired/1 -> Sum2/1
  pz/1(vzd) -> Sum/2
  z_desired/1 -> Sum4/1
  vz_desired/1 -> Sum/1
  Saturation1/1 -> phi/1
  Saturation2/1 -> theta/1
  psi/1 -> MATLAB Function/3(psi)
  py/1(vyd) -> Sum2/2
  MATLAB Function/1(phi) -> Saturation1/1
  MATLAB Function/2(theta) -> Saturation2/1
  "vx "/1(y) -> MATLAB Function/1(eax)
  "vy "/1(y) -> MATLAB Function/2(eay)
  az/1 -> Sum6/1
  vx/1 -> Sum7/3
  px/1(vxd) -> Sum7/2
  vx_desired/1 -> Sum7/1
  x_desired/1 -> Sum1/1

== system PosCtrl_tune/M300_00/Quadcopter Dynamics/六自由度模型 ==
  Mb : Inport
  f : Inport  Port=2
  Rigid-Body Dynamic Model : Subsystem
  "Rigid-Body Kinematic Model " : Subsystem
  "xe " : Outport  VectorParamsAs1DForOutWhenUnconnected=off
  ve : Outport  Port=2  VectorParamsAs1DForOutWhenUnconnected=off
  Euler : Outport  Port=3  VectorParamsAs1DForOutWhenUnconnected=off
  DCM : Outport  Port=4  VectorParamsAs1DForOutWhenUnconnected=off
  "vb " : Outport  Port=5  VectorParamsAs1DForOutWhenUnconnected=off
  "p,q,r " : Outport  Port=6  VectorParamsAs1DForOutWhenUnconnected=off
  wires:
  Rigid-Body Dynamic Model/1("p,q,r ") -> "Rigid-Body Kinematic Model "/1(pqr), "p,q,r "/1
  "Rigid-Body Kinematic Model "/1(Euler) -> Euler/1
  "Rigid-Body Kinematic Model "/3(DCM) -> Rigid-Body Dynamic Model/3(DCM), DCM/1
  Mb/1 -> Rigid-Body Dynamic Model/1(Mb)
  f/1 -> Rigid-Body Dynamic Model/2(f)
  Rigid-Body Dynamic Model/2(ve) -> "Rigid-Body Kinematic Model "/2(ve), ve/1
  Rigid-Body Dynamic Model/3("vb ") -> "vb "/1
  "Rigid-Body Kinematic Model "/2("xe ") -> "xe "/1

== system PosCtrl_tune/M300_00/Quadcopter Dynamics/控制效果模型 ==
  MotorRads : Inport
  mg : Inport  Port=2
  DCM : Inport  Port=3
  Vb : Inport  Port=4
  p.q,r : Inport  Port=5
  Add1 : Sum  Inputs=+++
  Add2 : Sum
  Add7 : Sum
  Constant1 : Constant  Value=ModelParam_uavCCm
  Constant3 : Constant  Value=ModelParam_rotorCt
  Constant4 : Constant  Value=ModelParam_rotorCm
  Constant5 : Constant  Value=ModelParam_uavR
  Constant7 : Constant  Value=ModelParam_uavCd
  Jrp : Constant  Value=ModelParam_motorJm
  Product : Product  Multiplication=Matrix(*)
  Propeller Model : MATLAB Function  TreatAsAtomicUnit=on
  Transpose : Math  Operator=transpose  SignedPower=on  SaturateOnIntegerOverflow=on
  Mb : Outport  VectorParamsAs1DForOutWhenUnconnected=off
  Fb : Outport  Port=2  VectorParamsAs1DForOutWhenUnconnected=off
  wires:
  Add2/1 -> Fb/1
  Constant3/1 -> Propeller Model/4(Ct)
  Propeller Model/2(Fd) -> Add7/2
  Add7/1 -> Add2/2
  Propeller Model/1(Fb) -> Add7/1
  Product/1 -> Add2/1
  mg/1 -> Product/2
  DCM/1 -> Transpose/1
  Constant7/1 -> Propeller Model/6(Cd)
  Vb/1 -> Propeller Model/5(Vb)
  Constant5/1 -> Propeller Model/2(R)
  Constant4/1 -> Propeller Model/3(Cm)
  MotorRads/1 -> Propeller Model/1(w)
  Transpose/1 -> Product/1
  Propeller Model/3(Mb) -> Add1/1
  Propeller Model/4(Md) -> Add1/2
  Add1/1 -> Mb/1
  p.q,r/1 -> Propeller Model/7(wb)
  Constant1/1 -> Propeller Model/8(Cdm)
  Jrp/1 -> Propeller Model/9(Jrp)
  Propeller Model/5(Ga) -> Add1/3

== system PosCtrl_tune/M300_00/Quadcopter Dynamics/电机动态模型 ==
  note: Motor Dynamic
      | w=1/(Ts+1)*wb
  note: No. 1 motor
      |
      |          Saturation             Throttle --> Motor Speed
  inPWMs : Inport
  Demux1 : Demux
  Motor_Dynamics_{1..4} (4 alike) : StateSpace  A=-1/ModelParam_motorT  C=1/ModelParam_motorT  D=0  InitialCondition=ModelInit_Rads*ModelParam_motorT
  Mux1 : Mux
  Signal_Saturation_{1..4} (4 alike) : Saturate  UpperLimit=1  LowerLimit=0
  Throttle To rads Gain _1 : Subsystem
  Throttle To rads Gain _2 : Subsystem
  Throttle To rads Gain _3 : Subsystem
  Throttle To rads Gain _4 : Subsystem
  MotorRads : Outport  VectorParamsAs1DForOutWhenUnconnected=off
  wires:
  Throttle To rads Gain _4/1(Out5) -> Motor_Dynamics_4/1
  Signal_Saturation_4/1 -> Throttle To rads Gain _4/1(In5)
  Signal_Saturation_3/1 -> Throttle To rads Gain _3/1(In5)
  Signal_Saturation_2/1 -> Throttle To rads Gain _2/1(In5)
  Motor_Dynamics_4/1 -> Mux1/4
  Motor_Dynamics_3/1 -> Mux1/3
  Motor_Dynamics_2/1 -> Mux1/2
  Motor_Dynamics_1/1 -> Mux1/1
  Signal_Saturation_1/1 -> Throttle To rads Gain _1/1(In5)
  Mux1/1 -> MotorRads/1
  Throttle To rads Gain _3/1(Out5) -> Motor_Dynamics_3/1
  Throttle To rads Gain _2/1(Out5) -> Motor_Dynamics_2/1
  Throttle To rads Gain _1/1(Out5) -> Motor_Dynamics_1/1
  inPWMs/1 -> Demux1/1
  Demux1/4 -> Signal_Saturation_4/1
  Demux1/3 -> Signal_Saturation_3/1
  Demux1/2 -> Signal_Saturation_2/1
  Demux1/1 -> Signal_Saturation_1/1

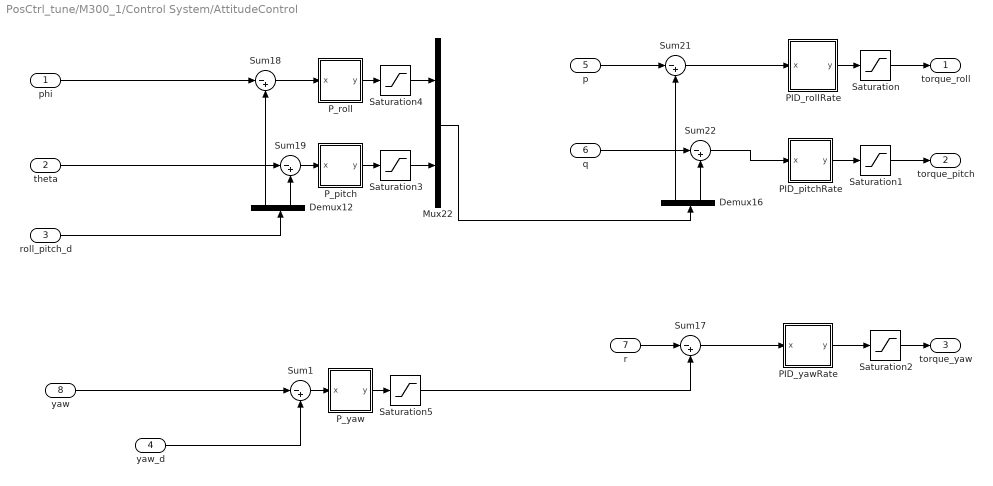
== system PosCtrl_tune/M300_1/Control System/AttitudeControl ==
  phi : Inport
  theta : Inport  Port=2
  roll_pitch_d : Inport  Port=3
  yaw_d : Inport  Port=4
  p : Inport  Port=5
  q : Inport  Port=6
  r : Inport  Port=7
  yaw : Inport  Port=8
  Demux12 : Demux  Outputs=2
  Demux16 : Demux  Outputs=2
  Mux22 : Mux  Inputs=2
  PID_pitchRate : Subsystem
  PID_rollRate : Subsystem
  PID_yawRate : Subsystem
  "P_pitch " : Subsystem
  "P_roll " : Subsystem
  P_yaw : Subsystem
  Saturation : Saturate  UpperLimit=1  LowerLimit=-1
  Saturation1 : Saturate  UpperLimit=1  LowerLimit=-1
  Saturation2 : Saturate
  Saturation3 : Saturate  UpperLimit=MAX_CONTROL_ANGLE_RATE_PITCH  LowerLimit=-MAX_CONTROL_ANGLE_RATE_PITCH
  Saturation4 : Saturate  UpperLimit=MAX_CONTROL_ANGLE_RATE_ROLL  LowerLimit=-MAX_CONTROL_ANGLE_RATE_ROLL
  Saturation5 : Saturate  UpperLimit=MAX_CONTROL_ANGLE_RATE_Y  LowerLimit=-MAX_CONTROL_ANGLE_RATE_Y
  Sum{1,17..19,21..22} (6 alike) : Sum  Inputs=|-+
  torque_roll : Outport  VectorParamsAs1DForOutWhenUnconnected=off
  torque_pitch : Outport  Port=2  VectorParamsAs1DForOutWhenUnconnected=off
  torque_yaw : Outport  Port=3  VectorParamsAs1DForOutWhenUnconnected=off
  wires:
  r/1 -> Sum17/1
  Sum19/1 -> "P_pitch "/1(x)
  "P_pitch "/1(y) -> Saturation3/1
  "P_roll "/1(y) -> Saturation4/1
  roll_pitch_d/1 -> Demux12/1
  Demux12/1 -> Sum18/2
  Demux12/2 -> Sum19/2
  phi/1 -> Sum18/1
  theta/1 -> Sum19/1
  Sum18/1 -> "P_roll "/1(x)
  Sum22/1 -> PID_pitchRate/1(x)
  Sum17/1 -> PID_yawRate/1(x)
  p/1 -> Sum21/1
  q/1 -> Sum22/1
  Sum21/1 -> PID_rollRate/1(x)
  Demux16/1 -> Sum21/2
  PID_pitchRate/1(y) -> Saturation1/1
  PID_rollRate/1(y) -> Saturation/1
  PID_yawRate/1(y) -> Saturation2/1
  Saturation/1 -> torque_roll/1
  Saturation1/1 -> torque_pitch/1
  Saturation2/1 -> torque_yaw/1
  Mux22/1 -> Demux16/1
  Saturation4/1 -> Mux22/1
  Saturation3/1 -> Mux22/2
  Demux16/2 -> Sum22/2
  Saturation5/1 -> Sum17/2
  Sum1/1 -> P_yaw/1(x)
  P_yaw/1(y) -> Saturation5/1
  yaw/1 -> Sum1/1
  yaw_d/1 -> Sum1/2

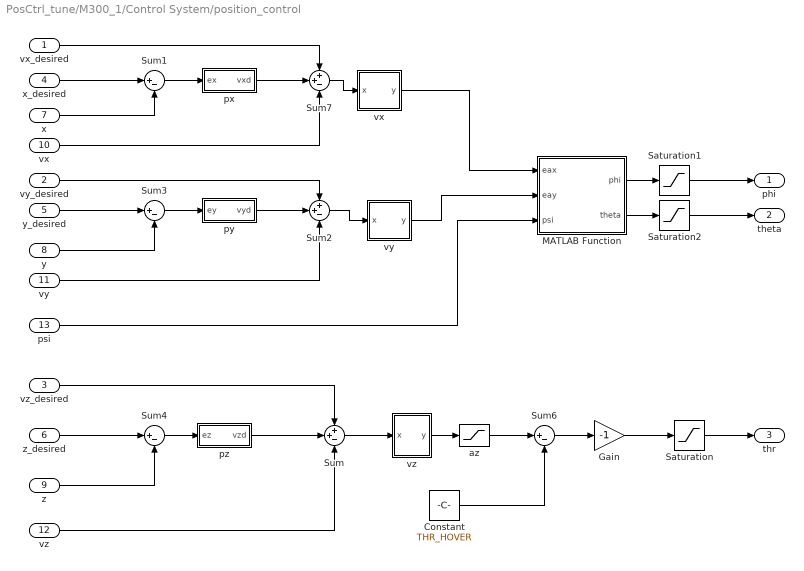
== system PosCtrl_tune/M300_1/Control System/position_control ==
  vx_desired : Inport
  vy_desired : Inport  Port=2
  vz_desired : Inport  Port=3
  x_desired : Inport  Port=4
  y_desired : Inport  Port=5
  z_desired : Inport  Port=6
  x : Inport  Port=7
  y : Inport  Port=8
  z : Inport  Port=9
  vx : Inport  Port=10
  vy : Inport  Port=11
  vz : Inport  Port=12
  psi : Inport  Port=13
  Constant : Constant  Value=THR_HOVER
  Gain : Gain  Gain=-1
  MATLAB Function : MATLAB Function  TreatAsAtomicUnit=on
  Saturation : Saturate  UpperLimit=MAX_MAN_THR  LowerLimit=0
  Saturation1 : Saturate  UpperLimit=MAX_CONTROL_ANGLE_ROLL*DEG2RAD  LowerLimit=-MAX_CONTROL_ANGLE_ROLL*DEG2RAD
  Saturation2 : Saturate  UpperLimit=MAX_CONTROL_ANGLE_PITCH*DEG2RAD  LowerLimit=-MAX_CONTROL_ANGLE_PITCH*DEG2RAD
  Sum : Sum  Inputs=++-
  Sum{1,3..4,6} (4 alike) : Sum  Inputs=|+-
  Sum2 : Sum  Inputs=++-
  Sum7 : Sum  Inputs=++-
  az : Saturate  UpperLimit=0.4  LowerLimit=-0.4
  px : Subsystem
  py : Subsystem
  pz : Subsystem
  "vx " : Subsystem
  "vy " : Subsystem
  "vz " : Subsystem
  phi : Outport  VectorParamsAs1DForOutWhenUnconnected=off
  theta : Outport  Port=2  VectorParamsAs1DForOutWhenUnconnected=off
  thr : Outport  Port=3  VectorParamsAs1DForOutWhenUnconnected=off
  wires:
  Saturation/1 -> thr/1
  Gain/1 -> Saturation/1
  Sum6/1 -> Gain/1
  "vz "/1(y) -> az/1
  Sum4/1 -> pz/1(ez)
  z/1 -> Sum4/2
  Constant/1 -> Sum6/2
  Sum/1 -> "vz "/1(x)
  vz/1 -> Sum/3
  x/1 -> Sum1/2
  y/1 -> Sum3/2
  Sum3/1 -> py/1(ey)
  y_desired/1 -> Sum3/1
  vy/1 -> Sum2/3
  Sum2/1 -> "vy "/1(x)
  Sum7/1 -> "vx "/1(x)
  Sum1/1 -> px/1(ex)
  vy_desired/1 -> Sum2/1
  pz/1(vzd) -> Sum/2
  z_desired/1 -> Sum4/1
  vz_desired/1 -> Sum/1
  Saturation1/1 -> phi/1
  Saturation2/1 -> theta/1
  psi/1 -> MATLAB Function/3(psi)
  py/1(vyd) -> Sum2/2
  MATLAB Function/1(phi) -> Saturation1/1
  MATLAB Function/2(theta) -> Saturation2/1
  "vx "/1(y) -> MATLAB Function/1(eax)
  "vy "/1(y) -> MATLAB Function/2(eay)
  az/1 -> Sum6/1
  vx/1 -> Sum7/3
  px/1(vxd) -> Sum7/2
  vx_desired/1 -> Sum7/1
  x_desired/1 -> Sum1/1

== system PosCtrl_tune/M300_1/Quadcopter Dynamics/六自由度模型 ==
  Mb : Inport
  f : Inport  Port=2
  Rigid-Body Dynamic Model : Subsystem
  "Rigid-Body Kinematic Model " : Subsystem
  "xe " : Outport  VectorParamsAs1DForOutWhenUnconnected=off
  ve : Outport  Port=2  VectorParamsAs1DForOutWhenUnconnected=off
  Euler : Outport  Port=3  VectorParamsAs1DForOutWhenUnconnected=off
  DCM : Outport  Port=4  VectorParamsAs1DForOutWhenUnconnected=off
  "vb " : Outport  Port=5  VectorParamsAs1DForOutWhenUnconnected=off
  "p,q,r " : Outport  Port=6  VectorParamsAs1DForOutWhenUnconnected=off
  wires:
  Rigid-Body Dynamic Model/1("p,q,r ") -> "Rigid-Body Kinematic Model "/1(pqr), "p,q,r "/1
  "Rigid-Body Kinematic Model "/1(Euler) -> Euler/1
  "Rigid-Body Kinematic Model "/3(DCM) -> Rigid-Body Dynamic Model/3(DCM), DCM/1
  Mb/1 -> Rigid-Body Dynamic Model/1(Mb)
  f/1 -> Rigid-Body Dynamic Model/2(f)
  Rigid-Body Dynamic Model/2(ve) -> "Rigid-Body Kinematic Model "/2(ve), ve/1
  Rigid-Body Dynamic Model/3("vb ") -> "vb "/1
  "Rigid-Body Kinematic Model "/2("xe ") -> "xe "/1

== system PosCtrl_tune/M300_1/Quadcopter Dynamics/控制效果模型 ==
  MotorRads : Inport
  mg : Inport  Port=2
  DCM : Inport  Port=3
  Vb : Inport  Port=4
  p.q,r : Inport  Port=5
  Add1 : Sum  Inputs=+++
  Add2 : Sum
  Add7 : Sum
  Constant1 : Constant  Value=ModelParam_uavCCm
  Constant3 : Constant  Value=ModelParam_rotorCt
  Constant4 : Constant  Value=ModelParam_rotorCm
  Constant5 : Constant  Value=ModelParam_uavR
  Constant7 : Constant  Value=ModelParam_uavCd
  Jrp : Constant  Value=ModelParam_motorJm
  Product : Product  Multiplication=Matrix(*)
  Propeller Model : MATLAB Function  TreatAsAtomicUnit=on
  Transpose : Math  Operator=transpose  SignedPower=on  SaturateOnIntegerOverflow=on
  Mb : Outport  VectorParamsAs1DForOutWhenUnconnected=off
  Fb : Outport  Port=2  VectorParamsAs1DForOutWhenUnconnected=off
  wires:
  Add2/1 -> Fb/1
  Constant3/1 -> Propeller Model/4(Ct)
  Propeller Model/2(Fd) -> Add7/2
  Add7/1 -> Add2/2
  Propeller Model/1(Fb) -> Add7/1
  Product/1 -> Add2/1
  mg/1 -> Product/2
  DCM/1 -> Transpose/1
  Constant7/1 -> Propeller Model/6(Cd)
  Vb/1 -> Propeller Model/5(Vb)
  Constant5/1 -> Propeller Model/2(R)
  Constant4/1 -> Propeller Model/3(Cm)
  MotorRads/1 -> Propeller Model/1(w)
  Transpose/1 -> Product/1
  Propeller Model/3(Mb) -> Add1/1
  Propeller Model/4(Md) -> Add1/2
  Add1/1 -> Mb/1
  p.q,r/1 -> Propeller Model/7(wb)
  Constant1/1 -> Propeller Model/8(Cdm)
  Jrp/1 -> Propeller Model/9(Jrp)
  Propeller Model/5(Ga) -> Add1/3

== system PosCtrl_tune/M300_1/Quadcopter Dynamics/电机动态模型 ==
  note: Motor Dynamic
      | w=1/(Ts+1)*wb
  note: No. 1 motor
      |
      |          Saturation             Throttle --> Motor Speed
  inPWMs : Inport
  Demux1 : Demux
  Motor_Dynamics_{1..4} (4 alike) : StateSpace  A=-1/ModelParam_motorT  C=1/ModelParam_motorT  D=0  InitialCondition=ModelInit_Rads*ModelParam_motorT
  Mux1 : Mux
  Signal_Saturation_{1..4} (4 alike) : Saturate  UpperLimit=1  LowerLimit=0
  Throttle To rads Gain _1 : Subsystem
  Throttle To rads Gain _2 : Subsystem
  Throttle To rads Gain _3 : Subsystem
  Throttle To rads Gain _4 : Subsystem
  MotorRads : Outport  VectorParamsAs1DForOutWhenUnconnected=off
  wires:
  Throttle To rads Gain _4/1(Out5) -> Motor_Dynamics_4/1
  Signal_Saturation_4/1 -> Throttle To rads Gain _4/1(In5)
  Signal_Saturation_3/1 -> Throttle To rads Gain _3/1(In5)
  Signal_Saturation_2/1 -> Throttle To rads Gain _2/1(In5)
  Motor_Dynamics_4/1 -> Mux1/4
  Motor_Dynamics_3/1 -> Mux1/3
  Motor_Dynamics_2/1 -> Mux1/2
  Motor_Dynamics_1/1 -> Mux1/1
  Signal_Saturation_1/1 -> Throttle To rads Gain _1/1(In5)
  Mux1/1 -> MotorRads/1
  Throttle To rads Gain _3/1(Out5) -> Motor_Dynamics_3/1
  Throttle To rads Gain _2/1(Out5) -> Motor_Dynamics_2/1
  Throttle To rads Gain _1/1(Out5) -> Motor_Dynamics_1/1
  inPWMs/1 -> Demux1/1
  Demux1/4 -> Signal_Saturation_4/1
  Demux1/3 -> Signal_Saturation_3/1
  Demux1/2 -> Signal_Saturation_2/1
  Demux1/1 -> Signal_Saturation_1/1

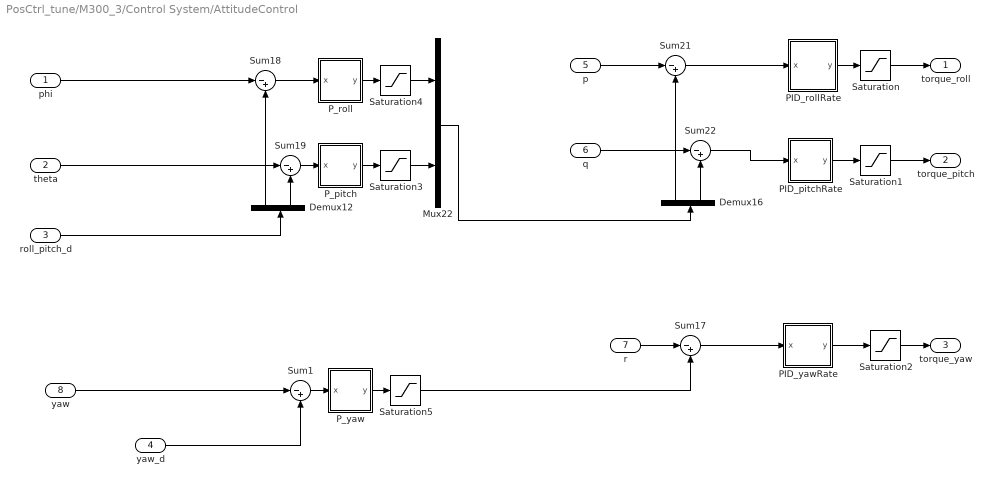
== system PosCtrl_tune/M300_3/Control System/AttitudeControl ==
  phi : Inport
  theta : Inport  Port=2
  roll_pitch_d : Inport  Port=3
  yaw_d : Inport  Port=4
  p : Inport  Port=5
  q : Inport  Port=6
  r : Inport  Port=7
  yaw : Inport  Port=8
  Demux12 : Demux  Outputs=2
  Demux16 : Demux  Outputs=2
  Mux22 : Mux  Inputs=2
  PID_pitchRate : Subsystem
  PID_rollRate : Subsystem
  PID_yawRate : Subsystem
  "P_pitch " : Subsystem
  "P_roll " : Subsystem
  P_yaw : Subsystem
  Saturation : Saturate  UpperLimit=1  LowerLimit=-1
  Saturation1 : Saturate  UpperLimit=1  LowerLimit=-1
  Saturation2 : Saturate
  Saturation3 : Saturate  UpperLimit=MAX_CONTROL_ANGLE_RATE_PITCH  LowerLimit=-MAX_CONTROL_ANGLE_RATE_PITCH
  Saturation4 : Saturate  UpperLimit=MAX_CONTROL_ANGLE_RATE_ROLL  LowerLimit=-MAX_CONTROL_ANGLE_RATE_ROLL
  Saturation5 : Saturate  UpperLimit=MAX_CONTROL_ANGLE_RATE_Y  LowerLimit=-MAX_CONTROL_ANGLE_RATE_Y
  Sum{1,17..19,21..22} (6 alike) : Sum  Inputs=|-+
  torque_roll : Outport  VectorParamsAs1DForOutWhenUnconnected=off
  torque_pitch : Outport  Port=2  VectorParamsAs1DForOutWhenUnconnected=off
  torque_yaw : Outport  Port=3  VectorParamsAs1DForOutWhenUnconnected=off
  wires:
  r/1 -> Sum17/1
  Sum19/1 -> "P_pitch "/1(x)
  "P_pitch "/1(y) -> Saturation3/1
  "P_roll "/1(y) -> Saturation4/1
  roll_pitch_d/1 -> Demux12/1
  Demux12/1 -> Sum18/2
  Demux12/2 -> Sum19/2
  phi/1 -> Sum18/1
  theta/1 -> Sum19/1
  Sum18/1 -> "P_roll "/1(x)
  Sum22/1 -> PID_pitchRate/1(x)
  Sum17/1 -> PID_yawRate/1(x)
  p/1 -> Sum21/1
  q/1 -> Sum22/1
  Sum21/1 -> PID_rollRate/1(x)
  Demux16/1 -> Sum21/2
  PID_pitchRate/1(y) -> Saturation1/1
  PID_rollRate/1(y) -> Saturation/1
  PID_yawRate/1(y) -> Saturation2/1
  Saturation/1 -> torque_roll/1
  Saturation1/1 -> torque_pitch/1
  Saturation2/1 -> torque_yaw/1
  Mux22/1 -> Demux16/1
  Saturation4/1 -> Mux22/1
  Saturation3/1 -> Mux22/2
  Demux16/2 -> Sum22/2
  Saturation5/1 -> Sum17/2
  Sum1/1 -> P_yaw/1(x)
  P_yaw/1(y) -> Saturation5/1
  yaw/1 -> Sum1/1
  yaw_d/1 -> Sum1/2

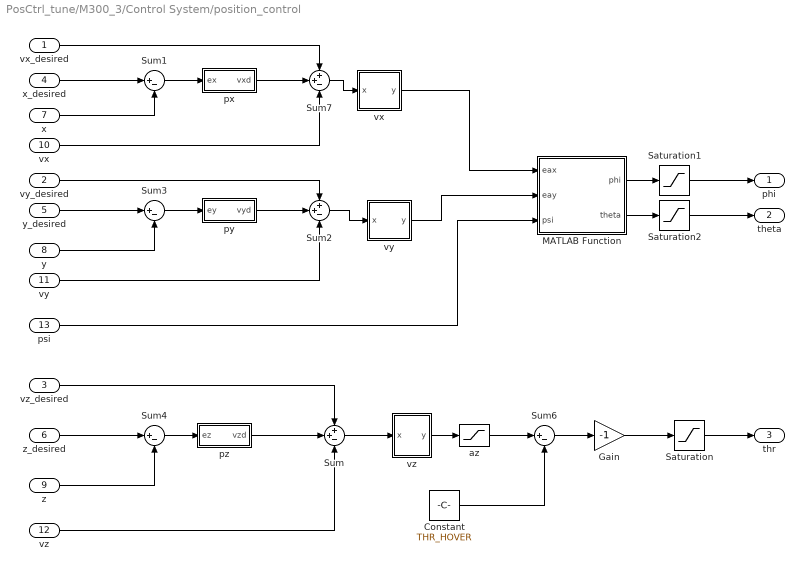
== system PosCtrl_tune/M300_3/Control System/position_control ==
  vx_desired : Inport
  vy_desired : Inport  Port=2
  vz_desired : Inport  Port=3
  x_desired : Inport  Port=4
  y_desired : Inport  Port=5
  z_desired : Inport  Port=6
  x : Inport  Port=7
  y : Inport  Port=8
  z : Inport  Port=9
  vx : Inport  Port=10
  vy : Inport  Port=11
  vz : Inport  Port=12
  psi : Inport  Port=13
  Constant : Constant  Value=THR_HOVER
  Gain : Gain  Gain=-1
  MATLAB Function : MATLAB Function  TreatAsAtomicUnit=on
  Saturation : Saturate  UpperLimit=MAX_MAN_THR  LowerLimit=0
  Saturation1 : Saturate  UpperLimit=MAX_CONTROL_ANGLE_ROLL*DEG2RAD  LowerLimit=-MAX_CONTROL_ANGLE_ROLL*DEG2RAD
  Saturation2 : Saturate  UpperLimit=MAX_CONTROL_ANGLE_PITCH*DEG2RAD  LowerLimit=-MAX_CONTROL_ANGLE_PITCH*DEG2RAD
  Sum : Sum  Inputs=++-
  Sum{1,3..4,6} (4 alike) : Sum  Inputs=|+-
  Sum2 : Sum  Inputs=++-
  Sum7 : Sum  Inputs=++-
  az : Saturate  UpperLimit=0.4  LowerLimit=-0.4
  px : Subsystem
  py : Subsystem
  pz : Subsystem
  "vx " : Subsystem
  "vy " : Subsystem
  "vz " : Subsystem
  phi : Outport  VectorParamsAs1DForOutWhenUnconnected=off
  theta : Outport  Port=2  VectorParamsAs1DForOutWhenUnconnected=off
  thr : Outport  Port=3  VectorParamsAs1DForOutWhenUnconnected=off
  wires:
  Saturation/1 -> thr/1
  Gain/1 -> Saturation/1
  Sum6/1 -> Gain/1
  "vz "/1(y) -> az/1
  Sum4/1 -> pz/1(ez)
  z/1 -> Sum4/2
  Constant/1 -> Sum6/2
  Sum/1 -> "vz "/1(x)
  vz/1 -> Sum/3
  x/1 -> Sum1/2
  y/1 -> Sum3/2
  Sum3/1 -> py/1(ey)
  y_desired/1 -> Sum3/1
  vy/1 -> Sum2/3
  Sum2/1 -> "vy "/1(x)
  Sum7/1 -> "vx "/1(x)
  Sum1/1 -> px/1(ex)
  vy_desired/1 -> Sum2/1
  pz/1(vzd) -> Sum/2
  z_desired/1 -> Sum4/1
  vz_desired/1 -> Sum/1
  Saturation1/1 -> phi/1
  Saturation2/1 -> theta/1
  psi/1 -> MATLAB Function/3(psi)
  py/1(vyd) -> Sum2/2
  MATLAB Function/1(phi) -> Saturation1/1
  MATLAB Function/2(theta) -> Saturation2/1
  "vx "/1(y) -> MATLAB Function/1(eax)
  "vy "/1(y) -> MATLAB Function/2(eay)
  az/1 -> Sum6/1
  vx/1 -> Sum7/3
  px/1(vxd) -> Sum7/2
  vx_desired/1 -> Sum7/1
  x_desired/1 -> Sum1/1

== system PosCtrl_tune/M300_3/M300_2/Control System ==
  xd : Inport
  yd : Inport  Port=2
  zd : Inport  Port=3
  yawRate_d : Inport  Port=4
  vxd : Inport  Port=5
  vyd : Inport  Port=6
  vzd : Inport  Port=7
  p : Inport  Port=8  PortDimensions=1
  q : Inport  Port=9  PortDimensions=1
  r : Inport  Port=10  PortDimensions=1
  roll : Inport  Port=11  PortDimensions=1
  pitch : Inport  Port=12  PortDimensions=1
  yaw : Inport  Port=13  PortDimensions=1
  x : Inport  Port=14
  y : Inport  Port=15
  z : Inport  Port=16
  vx : Inport  Port=17
  vy : Inport  Port=18
  vz : Inport  Port=19
  AttitudeControl : Subsystem
  Bus Creator : BusCreator  Inputs=2
  Mux12 : Mux
  Output_Limits1 : Saturate  UpperLimit=2000  LowerLimit=1000
  position_control : Subsystem
  pwm_out2 : MATLAB Function  SystemSampleTime=0.004
  PWM : Outport  VectorParamsAs1DForOutWhenUnconnected=off
  wires:
  Mux12/1 -> Output_Limits1/1
  AttitudeControl/2(torque_pitch) -> pwm_out2/2(Pitch)
  AttitudeControl/1(torque_roll) -> pwm_out2/1(Roll)
  pwm_out2/1(M1) -> Mux12/1
  pwm_out2/3(M3) -> Mux12/3
  pwm_out2/2(M2) -> Mux12/2
  AttitudeControl/3(torque_yaw) -> pwm_out2/3(Yaw)
  yawRate_d/1 -> AttitudeControl/4(yawRate_d)
  p/1 -> AttitudeControl/5(p)
  pwm_out2/4(M4) -> Mux12/4
  roll/1 -> AttitudeControl/1(phi)
  pitch/1 -> AttitudeControl/2(theta)
  position_control/1(phi) -> Bus Creator/1
  position_control/2(theta) -> Bus Creator/2
  Bus Creator/1 -> AttitudeControl/3(roll_pitch_d)
  position_control/3(thr) -> pwm_out2/4(Thrust)
  vxd/1 -> position_control/1(vx_desired)
  vyd/1 -> position_control/2(vy_desired)
  vzd/1 -> position_control/3(vz_desired)
  x/1 -> position_control/7(x)
  y/1 -> position_control/8(y)
  z/1 -> position_control/9(z)
  vx/1 -> position_control/10(vx)
  vy/1 -> position_control/11(vy)
  vz/1 -> position_control/12(vz)
  yaw/1 -> position_control/13(psi)
  Output_Limits1/1 -> PWM/1
  r/1 -> AttitudeControl/7(r)
  q/1 -> AttitudeControl/6(q)
  xd/1 -> position_control/4(x_desired)
  yd/1 -> position_control/5(y_desired)
  zd/1 -> position_control/6(z_desired)

== system PosCtrl_tune/M300_3/M300_2/Quadcopter Dynamics ==
  note: 输入为1000至2000的PWM信号，
      | 需要归一化为0~1。
  inPWMs : Inport
  Constant2 : Constant  Value=[1000,1000,1000,1000]
  Demux2 : Demux
  Gain : Gain  Gain=30/pi
  Gain1 : Gain  Gain=1/1000
  Gain2 : Gain  Gain=-1
  Gain3 : Gain  Gain=10
  Gain4 : Gain  Gain=-1
  Gain5 : Gain
  Gain6 : Gain
  Mux : Mux
  Product1 : Product
  Saturation : Saturate  UpperLimit=1  LowerLimit=0
  Sum : Sum  Inputs=|+-
  g : Constant  Value=[0,0,ModelParam_envGravityAcc]
  mass : Constant  Value=ModelParam_uavMass
  六自由度模型 : Subsystem
  控制效果模型 : Subsystem
  电机动态模型 : Subsystem
  PosE : Outport  VectorParamsAs1DForOutWhenUnconnected=off
  VelE : Outport  Port=2  VectorParamsAs1DForOutWhenUnconnected=off
  AngEuler : Outport  Port=3  VectorParamsAs1DForOutWhenUnconnected=off
  AngRateB : Outport  Port=4  VectorParamsAs1DForOutWhenUnconnected=off
  MotorRPMS : Outport  Port=5  VectorParamsAs1DForOutWhenUnconnected=off
  wires:
  Saturation/1 -> 电机动态模型/1(inPWMs)
  六自由度模型/6("p,q,r ") -> 控制效果模型/5(p.q,r), AngRateB/1
  mass/1 -> Product1/1
  六自由度模型/4(DCM) -> 控制效果模型/3(DCM)
  电机动态模型/1(MotorRads) -> Gain/1, 控制效果模型/1(MotorRads)
  Gain1/1 -> Saturation/1
  六自由度模型/2(ve) -> VelE/1
  Sum/1 -> Gain1/1
  Product1/1 -> 控制效果模型/2(mg)
  六自由度模型/5("vb ") -> 控制效果模型/4(Vb)
  六自由度模型/1("xe ") -> PosE/1
  六自由度模型/3(Euler) -> AngEuler/1
  控制效果模型/1(Mb) -> 六自由度模型/1(Mb)
  inPWMs/1 -> Sum/1
  控制效果模型/2(Fb) -> 六自由度模型/2(f)
  Constant2/1 -> Sum/2
  g/1 -> Product1/2
  Demux2/3 -> Gain4/1
  Demux2/4 -> Gain6/1
  Gain2/1 -> Mux/1
  Gain4/1 -> Mux/3
  Gain6/1 -> Mux/4
  Mux/1 -> Gain3/1
  Demux2/1 -> Gain2/1
  Gain5/1 -> Mux/2
  Demux2/2 -> Gain5/1
  Gain/1 -> Demux2/1
  Gain3/1 -> MotorRPMS/1
